simulink model "project_1"  (R2020b)
settings: Solver=VariableStepAuto  StartTime=0.0  StopTime=10.0  RelTol=1e-3
settings Model: Creator=shrin  LastModifiedBy=shrin

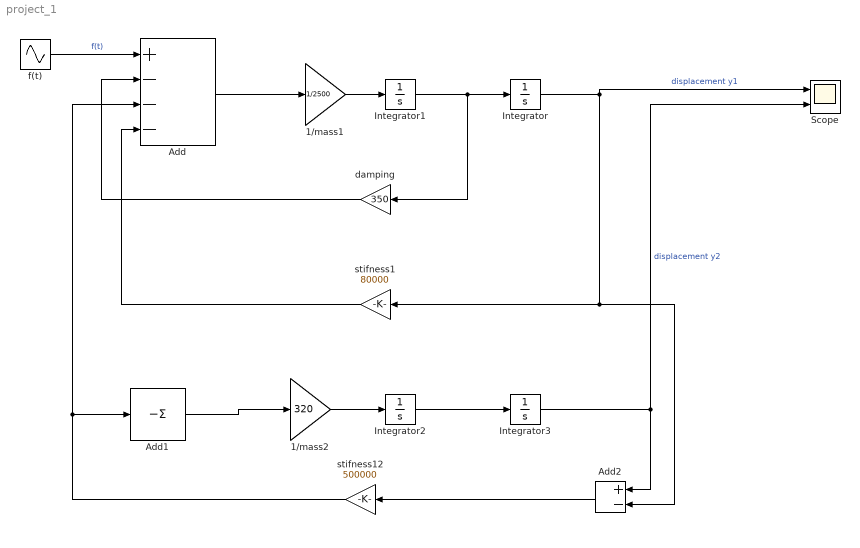
== system project_1 ==
  1/mass1 : Gain  Gain=1/2500
  1/mass2 : Gain  Gain=320
  Add : Sum  Inputs=+---
  Add1 : Sum  Inputs=-
  Add2 : Sum  Inputs=+-
  Integrator{,1..3} (4 alike) : Integrator
  Scope : Scope  NumInputPorts=2
  damping : Gain  Gain=350
  f(t) : Sin  Amplitude=2  Frequency=10  SampleTime=0
  stifness1 : Gain  Gain=80000
  stifness12 : Gain  Gain=500000
  wires:
  stifness12/1 -> Add1/1, Add/3
  Add1/1 -> 1/mass2/1
  Integrator2/1 -> Integrator3/1
  1/mass2/1 -> Integrator2/1
  Add2/1 -> stifness12/1
  Integrator1/1 -> damping/1, Integrator/1
  Integrator3/1 -> Scope/2, Add2/1  "displacement y2"
  Add/1 -> 1/mass1/1
  f(t)/1 -> Add/1  "f(t)"
  Integrator/1 -> Scope/1, Add2/2, stifness1/1  "displacement y1"
  damping/1 -> Add/2
  stifness1/1 -> Add/4
  1/mass1/1 -> Integrator1/1
